simulink model "c00011M_harness"  (R2018a)
settings: Solver=FixedStepAuto  StartTime=0.0  StopTime=300  FixedStep=0.1  RelTol=1e-3
undefined symbols (not defined in the file): A1, hmax, PriorityTank, R1, R2, sigbuilder_block
(part 20 of 73)

== system c00011M_harness/M164/Tank3 ==
  CT3 : Inport
  F3 : Inport  Port=2
  E3 : Inport  Port=3
  T3 : Inport  Port=4
  EB3 : Inport  Port=5
  LL1 : Inport  Port=6
  LL2 : Inport  Port=7
  Control : Subsystem
  Logical Operator : Logic  AllPortsSameDT=off  OutDataTypeStr=boolean
  MasterTankControl : Subsystem
  Memory : Memory
  Memory1 : Memory
  Memory2 : Memory
  TankModel : Subsystem
  LL3 : Outport
  wires:
  TankModel/1(LiquidLevel) -> Memory/1, LL3/1
  Control/1(LiquidIn) -> Logical Operator/1
  Control/2(LiquidOut) -> TankModel/2(LiquidOut)
  Memory/1 -> MasterTankControl/3(LiquidTank3), Control/5(LiquidLevel)
  CT3/1 -> Control/1(ControlType)
  F3/1 -> Control/2(Fill)
  E3/1 -> Control/3(Empty)
  LL2/1 -> Memory2/1
  Memory2/1 -> MasterTankControl/2(LiquidTank2)
  Memory1/1 -> MasterTankControl/1(LiquidTank1)
  EB3/1 -> Control/4(EmergencyButton)
  MasterTankControl/1(AllowTheTankFilling) -> Logical Operator/2
  Logical Operator/1 -> TankModel/1(LiquidIn)
  LL1/1 -> Memory1/1

== system c00011M_harness/M165/Tank1 ==
  CT1 : Inport
  MR1 : Inport  Port=2
  T1 : Inport  Port=3
  EB1 : Inport  Port=4
  LL2 : Inport  Port=5
  LL3 : Inport  Port=6
  Control : Subsystem
  Logical Operator : Logic  AllPortsSameDT=off  OutDataTypeStr=boolean
  MasterTankControl : Subsystem
  Memory : Memory
  Memory1 : Memory
  Memory2 : Memory
  TankModel : Subsystem
  LL1 : Outport
  wires:
  TankModel/1(LiquidLevel) -> Memory/1, LL1/1
  Control/1(LiquidIn) -> Logical Operator/1
  Control/2(LiquidOut) -> TankModel/2(LiquidOut)
  Memory/1 -> Control/5(LiquidLevel), MasterTankControl/1(LiquidTank1)
  MR1/1 -> Control/3(ManualReference)
  CT1/1 -> Control/2(StartMaintenance), Control/1(ControlType)
  LL3/1 -> Memory2/1
  Memory2/1 -> MasterTankControl/3(LiquidTank3)
  Memory1/1 -> MasterTankControl/2(LiquidTank2)
  EB1/1 -> Control/4(EmergencyButton)
  MasterTankControl/1(AllowTheTankFilling) -> Logical Operator/2
  Logical Operator/1 -> TankModel/1(LiquidIn)
  LL2/1 -> Memory1/1

== system c00011M_harness/M165/Tank2 ==
  CT2 : Inport
  MR2 : Inport  Port=2
  T2 : Inport  Port=3
  EB2 : Inport  Port=4
  LL1 : Inport  Port=5
  LL3 : Inport  Port=6
  Control : Subsystem
  Logical Operator : Logic  AllPortsSameDT=off  OutDataTypeStr=boolean
  MasterTankControl : Subsystem
  Memory : Memory
  Memory1 : Memory
  Memory2 : Memory
  TankModel : Subsystem
  LL2 : Outport
  wires:
  TankModel/1(LiquidLevel) -> Memory/1, LL2/1
  Control/1(LiquidIn) -> Logical Operator/1
  Control/2(LiquidOut) -> TankModel/2(LiquidOut)
  Memory/1 -> Control/5(LiquidLevel), MasterTankControl/2(LiquidTank2)
  MR2/1 -> Control/3(ManualReference)
  CT2/1 -> Control/2(StartMaintenance), Control/1(ControlType)
  LL3/1 -> Memory2/1
  Memory2/1 -> MasterTankControl/3(LiquidTank3)
  Memory1/1 -> MasterTankControl/1(LiquidTank1)
  EB2/1 -> Control/4(EmergencyButton)
  MasterTankControl/1(AllowTheTankFilling) -> Logical Operator/2
  Logical Operator/1 -> TankModel/1(LiquidIn)
  LL1/1 -> Memory1/1

== system c00011M_harness/M165/Tank3 ==
  CT3 : Inport
  F3 : Inport  Port=2
  E3 : Inport  Port=3
  T3 : Inport  Port=4
  EB3 : Inport  Port=5
  LL1 : Inport  Port=6
  LL2 : Inport  Port=7
  Control : Subsystem
  Logical Operator : Logic  AllPortsSameDT=off  OutDataTypeStr=boolean
  MasterTankControl : Subsystem
  Memory : Memory
  Memory1 : Memory
  Memory2 : Memory
  TankModel : Subsystem
  LL3 : Outport
  wires:
  TankModel/1(LiquidLevel) -> Memory/1, LL3/1
  Control/1(LiquidIn) -> Logical Operator/1
  Control/2(LiquidOut) -> TankModel/2(LiquidOut)
  Memory/1 -> MasterTankControl/3(LiquidTank3), Control/5(LiquidLevel)
  CT3/1 -> Control/1(ControlType)
  F3/1 -> Control/2(Fill)
  E3/1 -> Control/3(Empty)
  LL2/1 -> Memory2/1
  Memory2/1 -> MasterTankControl/2(LiquidTank2)
  Memory1/1 -> MasterTankControl/1(LiquidTank1)
  EB3/1 -> Control/4(EmergencyButton)
  MasterTankControl/1(AllowTheTankFilling) -> Logical Operator/2
  Logical Operator/1 -> TankModel/1(LiquidIn)
  LL1/1 -> Memory1/1

== system c00011M_harness/M200/Tank1 ==
  CT1 : Inport
  MR1 : Inport  Port=2
  T1 : Inport  Port=3
  EB1 : Inport  Port=4
  LL2 : Inport  Port=5
  LL3 : Inport  Port=6
  Control : Subsystem
  Logical Operator : Logic  AllPortsSameDT=off  OutDataTypeStr=boolean
  MasterTankControl : Subsystem
  Memory : Memory
  Memory1 : Memory
  Memory2 : Memory
  TankModel : Subsystem
  LL1 : Outport
  wires:
  TankModel/1(LiquidLevel) -> Memory/1, LL1/1
  Control/1(LiquidIn) -> Logical Operator/1
  Control/2(LiquidOut) -> TankModel/2(LiquidOut)
  Memory/1 -> Control/5(LiquidLevel), MasterTankControl/1(LiquidTank1)
  MR1/1 -> Control/3(ManualReference)
  CT1/1 -> Control/2(StartMaintenance), Control/1(ControlType)
  LL3/1 -> Memory2/1
  Memory2/1 -> MasterTankControl/3(LiquidTank3)
  Memory1/1 -> MasterTankControl/2(LiquidTank2)
  EB1/1 -> Control/4(EmergencyButton)
  MasterTankControl/1(AllowTheTankFilling) -> Logical Operator/2
  Logical Operator/1 -> TankModel/1(LiquidIn)
  LL2/1 -> Memory1/1

== system c00011M_harness/M200/Tank2 ==
  CT2 : Inport
  MR2 : Inport  Port=2
  T2 : Inport  Port=3
  EB2 : Inport  Port=4
  LL1 : Inport  Port=5
  LL3 : Inport  Port=6
  Control : Subsystem
  Logical Operator : Logic  AllPortsSameDT=off  OutDataTypeStr=boolean
  MasterTankControl : Subsystem
  Memory : Memory
  Memory1 : Memory
  Memory2 : Memory
  TankModel : Subsystem
  LL2 : Outport
  wires:
  TankModel/1(LiquidLevel) -> Memory/1, LL2/1
  Control/1(LiquidIn) -> Logical Operator/1
  Control/2(LiquidOut) -> TankModel/2(LiquidOut)
  Memory/1 -> Control/5(LiquidLevel), MasterTankControl/2(LiquidTank2)
  MR2/1 -> Control/3(ManualReference)
  CT2/1 -> Control/2(StartMaintenance), Control/1(ControlType)
  LL3/1 -> Memory2/1
  Memory2/1 -> MasterTankControl/3(LiquidTank3)
  Memory1/1 -> MasterTankControl/1(LiquidTank1)
  EB2/1 -> Control/4(EmergencyButton)
  MasterTankControl/1(AllowTheTankFilling) -> Logical Operator/2
  Logical Operator/1 -> TankModel/1(LiquidIn)
  LL1/1 -> Memory1/1

== system c00011M_harness/M200/Tank3 ==
  CT3 : Inport
  F3 : Inport  Port=2
  E3 : Inport  Port=3
  T3 : Inport  Port=4
  EB3 : Inport  Port=5
  LL1 : Inport  Port=6
  LL2 : Inport  Port=7
  Control : Subsystem
  Logical Operator : Logic  AllPortsSameDT=off  OutDataTypeStr=boolean
  MasterTankControl : Subsystem
  Memory : Memory
  Memory1 : Memory
  Memory2 : Memory
  TankModel : Subsystem
  LL3 : Outport
  wires:
  TankModel/1(LiquidLevel) -> Memory/1, LL3/1
  Control/1(LiquidIn) -> Logical Operator/1
  Control/2(LiquidOut) -> TankModel/2(LiquidOut)
  Memory/1 -> MasterTankControl/3(LiquidTank3), Control/5(LiquidLevel)
  CT3/1 -> Control/1(ControlType)
  F3/1 -> Control/2(Fill)
  E3/1 -> Control/3(Empty)
  LL2/1 -> Memory2/1
  Memory2/1 -> MasterTankControl/2(LiquidTank2)
  Memory1/1 -> MasterTankControl/1(LiquidTank1)
  EB3/1 -> Control/4(EmergencyButton)
  MasterTankControl/1(AllowTheTankFilling) -> Logical Operator/2
  Logical Operator/1 -> TankModel/1(LiquidIn)
  LL1/1 -> Memory1/1

== system c00011M_harness/M201/Tank1 ==
  CT1 : Inport
  MR1 : Inport  Port=2
  T1 : Inport  Port=3
  EB1 : Inport  Port=4
  LL2 : Inport  Port=5
  LL3 : Inport  Port=6
  Control : Subsystem
  Logical Operator : Logic  AllPortsSameDT=off  OutDataTypeStr=boolean
  MasterTankControl : Subsystem
  Memory : Memory
  Memory1 : Memory
  Memory2 : Memory
  TankModel : Subsystem
  LL1 : Outport
  wires:
  TankModel/1(LiquidLevel) -> Memory/1, LL1/1
  Control/1(LiquidIn) -> Logical Operator/1
  Control/2(LiquidOut) -> TankModel/2(LiquidOut)
  Memory/1 -> Control/5(LiquidLevel), MasterTankControl/1(LiquidTank1)
  MR1/1 -> Control/3(ManualReference)
  CT1/1 -> Control/2(StartMaintenance), Control/1(ControlType)
  LL3/1 -> Memory2/1
  Memory2/1 -> MasterTankControl/3(LiquidTank3)
  Memory1/1 -> MasterTankControl/2(LiquidTank2)
  EB1/1 -> Control/4(EmergencyButton)
  MasterTankControl/1(AllowTheTankFilling) -> Logical Operator/2
  Logical Operator/1 -> TankModel/1(LiquidIn)
  LL2/1 -> Memory1/1

== system c00011M_harness/M201/Tank2 ==
  CT2 : Inport
  MR2 : Inport  Port=2
  T2 : Inport  Port=3
  EB2 : Inport  Port=4
  LL1 : Inport  Port=5
  LL3 : Inport  Port=6
  Control : Subsystem
  Logical Operator : Logic  AllPortsSameDT=off  OutDataTypeStr=boolean
  MasterTankControl : Subsystem
  Memory : Memory
  Memory1 : Memory
  Memory2 : Memory
  TankModel : Subsystem
  LL2 : Outport
  wires:
  TankModel/1(LiquidLevel) -> Memory/1, LL2/1
  Control/1(LiquidIn) -> Logical Operator/1
  Control/2(LiquidOut) -> TankModel/2(LiquidOut)
  Memory/1 -> Control/5(LiquidLevel), MasterTankControl/2(LiquidTank2)
  MR2/1 -> Control/3(ManualReference)
  CT2/1 -> Control/2(StartMaintenance), Control/1(ControlType)
  LL3/1 -> Memory2/1
  Memory2/1 -> MasterTankControl/3(LiquidTank3)
  Memory1/1 -> MasterTankControl/1(LiquidTank1)
  EB2/1 -> Control/4(EmergencyButton)
  MasterTankControl/1(AllowTheTankFilling) -> Logical Operator/2
  Logical Operator/1 -> TankModel/1(LiquidIn)
  LL1/1 -> Memory1/1

== system c00011M_harness/M201/Tank3 ==
  CT3 : Inport
  F3 : Inport  Port=2
  E3 : Inport  Port=3
  T3 : Inport  Port=4
  EB3 : Inport  Port=5
  LL1 : Inport  Port=6
  LL2 : Inport  Port=7
  Control : Subsystem
  Logical Operator : Logic  AllPortsSameDT=off  OutDataTypeStr=boolean
  MasterTankControl : Subsystem
  Memory : Memory
  Memory1 : Memory
  Memory2 : Memory
  TankModel : Subsystem
  LL3 : Outport
  wires:
  TankModel/1(LiquidLevel) -> Memory/1, LL3/1
  Control/1(LiquidIn) -> Logical Operator/1
  Control/2(LiquidOut) -> TankModel/2(LiquidOut)
  Memory/1 -> MasterTankControl/3(LiquidTank3), Control/5(LiquidLevel)
  CT3/1 -> Control/1(ControlType)
  F3/1 -> Control/2(Fill)
  E3/1 -> Control/3(Empty)
  LL2/1 -> Memory2/1
  Memory2/1 -> MasterTankControl/2(LiquidTank2)
  Memory1/1 -> MasterTankControl/1(LiquidTank1)
  EB3/1 -> Control/4(EmergencyButton)
  MasterTankControl/1(AllowTheTankFilling) -> Logical Operator/2
  Logical Operator/1 -> TankModel/1(LiquidIn)
  LL1/1 -> Memory1/1

== system c00011M_harness/M202/Tank1 ==
  CT1 : Inport
  MR1 : Inport  Port=2
  T1 : Inport  Port=3
  EB1 : Inport  Port=4
  LL2 : Inport  Port=5
  LL3 : Inport  Port=6
  Control : Subsystem
  Logical Operator : Logic  AllPortsSameDT=off  OutDataTypeStr=boolean
  MasterTankControl : Subsystem
  Memory : Memory
  Memory1 : Memory
  Memory2 : Memory
  TankModel : Subsystem
  LL1 : Outport
  wires:
  TankModel/1(LiquidLevel) -> Memory/1, LL1/1
  Control/1(LiquidIn) -> Logical Operator/1
  Control/2(LiquidOut) -> TankModel/2(LiquidOut)
  Memory/1 -> Control/5(LiquidLevel), MasterTankControl/1(LiquidTank1)
  MR1/1 -> Control/3(ManualReference)
  CT1/1 -> Control/2(StartMaintenance), Control/1(ControlType)
  LL3/1 -> Memory2/1
  Memory2/1 -> MasterTankControl/3(LiquidTank3)
  Memory1/1 -> MasterTankControl/2(LiquidTank2)
  EB1/1 -> Control/4(EmergencyButton)
  MasterTankControl/1(AllowTheTankFilling) -> Logical Operator/2
  Logical Operator/1 -> TankModel/1(LiquidIn)
  LL2/1 -> Memory1/1

== system c00011M_harness/M202/Tank2 ==
  CT2 : Inport
  MR2 : Inport  Port=2
  T2 : Inport  Port=3
  EB2 : Inport  Port=4
  LL1 : Inport  Port=5
  LL3 : Inport  Port=6
  Control : Subsystem
  Logical Operator : Logic  AllPortsSameDT=off  OutDataTypeStr=boolean
  MasterTankControl : Subsystem
  Memory : Memory
  Memory1 : Memory
  Memory2 : Memory
  TankModel : Subsystem
  LL2 : Outport
  wires:
  TankModel/1(LiquidLevel) -> Memory/1, LL2/1
  Control/1(LiquidIn) -> Logical Operator/1
  Control/2(LiquidOut) -> TankModel/2(LiquidOut)
  Memory/1 -> Control/5(LiquidLevel), MasterTankControl/2(LiquidTank2)
  MR2/1 -> Control/3(ManualReference)
  CT2/1 -> Control/2(StartMaintenance), Control/1(ControlType)
  LL3/1 -> Memory2/1
  Memory2/1 -> MasterTankControl/3(LiquidTank3)
  Memory1/1 -> MasterTankControl/1(LiquidTank1)
  EB2/1 -> Control/4(EmergencyButton)
  MasterTankControl/1(AllowTheTankFilling) -> Logical Operator/2
  Logical Operator/1 -> TankModel/1(LiquidIn)
  LL1/1 -> Memory1/1

== system c00011M_harness/M202/Tank3 ==
  CT3 : Inport
  F3 : Inport  Port=2
  E3 : Inport  Port=3
  T3 : Inport  Port=4
  EB3 : Inport  Port=5
  LL1 : Inport  Port=6
  LL2 : Inport  Port=7
  Control : Subsystem
  Logical Operator : Logic  AllPortsSameDT=off  OutDataTypeStr=boolean
  MasterTankControl : Subsystem
  Memory : Memory
  Memory1 : Memory
  Memory2 : Memory
  TankModel : Subsystem
  LL3 : Outport
  wires:
  TankModel/1(LiquidLevel) -> Memory/1, LL3/1
  Control/1(LiquidIn) -> Logical Operator/1
  Control/2(LiquidOut) -> TankModel/2(LiquidOut)
  Memory/1 -> MasterTankControl/3(LiquidTank3), Control/5(LiquidLevel)
  CT3/1 -> Control/1(ControlType)
  F3/1 -> Control/2(Fill)
  E3/1 -> Control/3(Empty)
  LL2/1 -> Memory2/1
  Memory2/1 -> MasterTankControl/2(LiquidTank2)
  Memory1/1 -> MasterTankControl/1(LiquidTank1)
  EB3/1 -> Control/4(EmergencyButton)
  MasterTankControl/1(AllowTheTankFilling) -> Logical Operator/2
  Logical Operator/1 -> TankModel/1(LiquidIn)
  LL1/1 -> Memory1/1

== system c00011M_harness/M203/Tank1 ==
  CT1 : Inport
  MR1 : Inport  Port=2
  T1 : Inport  Port=3
  EB1 : Inport  Port=4
  LL2 : Inport  Port=5
  LL3 : Inport  Port=6
  Control : Subsystem
  Logical Operator : Logic  AllPortsSameDT=off  OutDataTypeStr=boolean
  MasterTankControl : Subsystem
  Memory : Memory
  Memory1 : Memory
  Memory2 : Memory
  TankModel : Subsystem
  LL1 : Outport
  wires:
  TankModel/1(LiquidLevel) -> Memory/1, LL1/1
  Control/1(LiquidIn) -> Logical Operator/1
  Control/2(LiquidOut) -> TankModel/2(LiquidOut)
  Memory/1 -> Control/5(LiquidLevel), MasterTankControl/1(LiquidTank1)
  MR1/1 -> Control/3(ManualReference)
  CT1/1 -> Control/2(StartMaintenance), Control/1(ControlType)
  LL3/1 -> Memory2/1
  Memory2/1 -> MasterTankControl/3(LiquidTank3)
  Memory1/1 -> MasterTankControl/2(LiquidTank2)
  EB1/1 -> Control/4(EmergencyButton)
  MasterTankControl/1(AllowTheTankFilling) -> Logical Operator/2
  Logical Operator/1 -> TankModel/1(LiquidIn)
  LL2/1 -> Memory1/1

== system c00011M_harness/M203/Tank2 ==
  CT2 : Inport
  MR2 : Inport  Port=2
  T2 : Inport  Port=3
  EB2 : Inport  Port=4
  LL1 : Inport  Port=5
  LL3 : Inport  Port=6
  Control : Subsystem
  Logical Operator : Logic  AllPortsSameDT=off  OutDataTypeStr=boolean
  MasterTankControl : Subsystem
  Memory : Memory
  Memory1 : Memory
  Memory2 : Memory
  TankModel : Subsystem
  LL2 : Outport
  wires:
  TankModel/1(LiquidLevel) -> Memory/1, LL2/1
  Control/1(LiquidIn) -> Logical Operator/1
  Control/2(LiquidOut) -> TankModel/2(LiquidOut)
  Memory/1 -> Control/5(LiquidLevel), MasterTankControl/2(LiquidTank2)
  MR2/1 -> Control/3(ManualReference)
  CT2/1 -> Control/2(StartMaintenance), Control/1(ControlType)
  LL3/1 -> Memory2/1
  Memory2/1 -> MasterTankControl/3(LiquidTank3)
  Memory1/1 -> MasterTankControl/1(LiquidTank1)
  EB2/1 -> Control/4(EmergencyButton)
  MasterTankControl/1(AllowTheTankFilling) -> Logical Operator/2
  Logical Operator/1 -> TankModel/1(LiquidIn)
  LL1/1 -> Memory1/1

== system c00011M_harness/M203/Tank3 ==
  CT3 : Inport
  F3 : Inport  Port=2
  E3 : Inport  Port=3
  T3 : Inport  Port=4
  EB3 : Inport  Port=5
  LL1 : Inport  Port=6
  LL2 : Inport  Port=7
  Control : Subsystem
  Logical Operator : Logic  AllPortsSameDT=off  OutDataTypeStr=boolean
  MasterTankControl : Subsystem
  Memory : Memory
  Memory1 : Memory
  Memory2 : Memory
  TankModel : Subsystem
  LL3 : Outport
  wires:
  TankModel/1(LiquidLevel) -> Memory/1, LL3/1
  Control/1(LiquidIn) -> Logical Operator/1
  Control/2(LiquidOut) -> TankModel/2(LiquidOut)
  Memory/1 -> MasterTankControl/3(LiquidTank3), Control/5(LiquidLevel)
  CT3/1 -> Control/1(ControlType)
  F3/1 -> Control/2(Fill)
  E3/1 -> Control/3(Empty)
  LL2/1 -> Memory2/1
  Memory2/1 -> MasterTankControl/2(LiquidTank2)
  Memory1/1 -> MasterTankControl/1(LiquidTank1)
  EB3/1 -> Control/4(EmergencyButton)
  MasterTankControl/1(AllowTheTankFilling) -> Logical Operator/2
  Logical Operator/1 -> TankModel/1(LiquidIn)
  LL1/1 -> Memory1/1

== system c00011M_harness/M204/Tank1 ==
  CT1 : Inport
  MR1 : Inport  Port=2
  T1 : Inport  Port=3
  EB1 : Inport  Port=4
  LL2 : Inport  Port=5
  LL3 : Inport  Port=6
  Control : Subsystem
  Logical Operator : Logic  AllPortsSameDT=off  OutDataTypeStr=boolean
  MasterTankControl : Subsystem
  Memory : Memory
  Memory1 : Memory
  Memory2 : Memory
  TankModel : Subsystem
  LL1 : Outport
  wires:
  TankModel/1(LiquidLevel) -> Memory/1, LL1/1
  Control/1(LiquidIn) -> Logical Operator/1
  Control/2(LiquidOut) -> TankModel/2(LiquidOut)
  Memory/1 -> Control/5(LiquidLevel), MasterTankControl/1(LiquidTank1)
  MR1/1 -> Control/3(ManualReference)
  CT1/1 -> Control/2(StartMaintenance), Control/1(ControlType)
  LL3/1 -> Memory2/1
  Memory2/1 -> MasterTankControl/3(LiquidTank3)
  Memory1/1 -> MasterTankControl/2(LiquidTank2)
  EB1/1 -> Control/4(EmergencyButton)
  MasterTankControl/1(AllowTheTankFilling) -> Logical Operator/2
  Logical Operator/1 -> TankModel/1(LiquidIn)
  LL2/1 -> Memory1/1

== system c00011M_harness/M204/Tank2 ==
  CT2 : Inport
  MR2 : Inport  Port=2
  T2 : Inport  Port=3
  EB2 : Inport  Port=4
  LL1 : Inport  Port=5
  LL3 : Inport  Port=6
  Control : Subsystem
  Logical Operator : Logic  AllPortsSameDT=off  OutDataTypeStr=boolean
  MasterTankControl : Subsystem
  Memory : Memory
  Memory1 : Memory
  Memory2 : Memory
  TankModel : Subsystem
  LL2 : Outport
  wires:
  TankModel/1(LiquidLevel) -> Memory/1, LL2/1
  Control/1(LiquidIn) -> Logical Operator/1
  Control/2(LiquidOut) -> TankModel/2(LiquidOut)
  Memory/1 -> Control/5(LiquidLevel), MasterTankControl/2(LiquidTank2)
  MR2/1 -> Control/3(ManualReference)
  CT2/1 -> Control/2(StartMaintenance), Control/1(ControlType)
  LL3/1 -> Memory2/1
  Memory2/1 -> MasterTankControl/3(LiquidTank3)
  Memory1/1 -> MasterTankControl/1(LiquidTank1)
  EB2/1 -> Control/4(EmergencyButton)
  MasterTankControl/1(AllowTheTankFilling) -> Logical Operator/2
  Logical Operator/1 -> TankModel/1(LiquidIn)
  LL1/1 -> Memory1/1

== system c00011M_harness/M204/Tank3 ==
  CT3 : Inport
  F3 : Inport  Port=2
  E3 : Inport  Port=3
  T3 : Inport  Port=4
  EB3 : Inport  Port=5
  LL1 : Inport  Port=6
  LL2 : Inport  Port=7
  Control : Subsystem
  Logical Operator : Logic  AllPortsSameDT=off  OutDataTypeStr=boolean
  MasterTankControl : Subsystem
  Memory : Memory
  Memory1 : Memory
  Memory2 : Memory
  TankModel : Subsystem
  LL3 : Outport
  wires:
  TankModel/1(LiquidLevel) -> Memory/1, LL3/1
  Control/1(LiquidIn) -> Logical Operator/1
  Control/2(LiquidOut) -> TankModel/2(LiquidOut)
  Memory/1 -> MasterTankControl/3(LiquidTank3), Control/5(LiquidLevel)
  CT3/1 -> Control/1(ControlType)
  F3/1 -> Control/2(Fill)
  E3/1 -> Control/3(Empty)
  LL2/1 -> Memory2/1
  Memory2/1 -> MasterTankControl/2(LiquidTank2)
  Memory1/1 -> MasterTankControl/1(LiquidTank1)
  EB3/1 -> Control/4(EmergencyButton)
  MasterTankControl/1(AllowTheTankFilling) -> Logical Operator/2
  Logical Operator/1 -> TankModel/1(LiquidIn)
  LL1/1 -> Memory1/1

== system c00011M_harness/M205/Tank1 ==
  CT1 : Inport
  MR1 : Inport  Port=2
  T1 : Inport  Port=3
  EB1 : Inport  Port=4
  LL2 : Inport  Port=5
  LL3 : Inport  Port=6
  Control : Subsystem
  Logical Operator : Logic  AllPortsSameDT=off  OutDataTypeStr=boolean
  MasterTankControl : Subsystem
  Memory : Memory
  Memory1 : Memory
  Memory2 : Memory
  TankModel : Subsystem
  LL1 : Outport
  wires:
  TankModel/1(LiquidLevel) -> Memory/1, LL1/1
  Control/1(LiquidIn) -> Logical Operator/1
  Control/2(LiquidOut) -> TankModel/2(LiquidOut)
  Memory/1 -> Control/5(LiquidLevel), MasterTankControl/1(LiquidTank1)
  MR1/1 -> Control/3(ManualReference)
  CT1/1 -> Control/2(StartMaintenance), Control/1(ControlType)
  LL3/1 -> Memory2/1
  Memory2/1 -> MasterTankControl/3(LiquidTank3)
  Memory1/1 -> MasterTankControl/2(LiquidTank2)
  EB1/1 -> Control/4(EmergencyButton)
  MasterTankControl/1(AllowTheTankFilling) -> Logical Operator/2
  Logical Operator/1 -> TankModel/1(LiquidIn)
  LL2/1 -> Memory1/1

== system c00011M_harness/M205/Tank2 ==
  CT2 : Inport
  MR2 : Inport  Port=2
  T2 : Inport  Port=3
  EB2 : Inport  Port=4
  LL1 : Inport  Port=5
  LL3 : Inport  Port=6
  Control : Subsystem
  Logical Operator : Logic  AllPortsSameDT=off  OutDataTypeStr=boolean
  MasterTankControl : Subsystem
  Memory : Memory
  Memory1 : Memory
  Memory2 : Memory
  TankModel : Subsystem
  LL2 : Outport
  wires:
  TankModel/1(LiquidLevel) -> Memory/1, LL2/1
  Control/1(LiquidIn) -> Logical Operator/1
  Control/2(LiquidOut) -> TankModel/2(LiquidOut)
  Memory/1 -> Control/5(LiquidLevel), MasterTankControl/2(LiquidTank2)
  MR2/1 -> Control/3(ManualReference)
  CT2/1 -> Control/2(StartMaintenance), Control/1(ControlType)
  LL3/1 -> Memory2/1
  Memory2/1 -> MasterTankControl/3(LiquidTank3)
  Memory1/1 -> MasterTankControl/1(LiquidTank1)
  EB2/1 -> Control/4(EmergencyButton)
  MasterTankControl/1(AllowTheTankFilling) -> Logical Operator/2
  Logical Operator/1 -> TankModel/1(LiquidIn)
  LL1/1 -> Memory1/1

== system c00011M_harness/M205/Tank3 ==
  CT3 : Inport
  F3 : Inport  Port=2
  E3 : Inport  Port=3
  T3 : Inport  Port=4
  EB3 : Inport  Port=5
  LL1 : Inport  Port=6
  LL2 : Inport  Port=7
  Control : Subsystem
  Logical Operator : Logic  AllPortsSameDT=off  OutDataTypeStr=boolean
  MasterTankControl : Subsystem
  Memory : Memory
  Memory1 : Memory
  Memory2 : Memory
  TankModel : Subsystem
  LL3 : Outport
  wires:
  TankModel/1(LiquidLevel) -> Memory/1, LL3/1
  Control/1(LiquidIn) -> Logical Operator/1
  Control/2(LiquidOut) -> TankModel/2(LiquidOut)
  Memory/1 -> MasterTankControl/3(LiquidTank3), Control/5(LiquidLevel)
  CT3/1 -> Control/1(ControlType)
  F3/1 -> Control/2(Fill)
  E3/1 -> Control/3(Empty)
  LL2/1 -> Memory2/1
  Memory2/1 -> MasterTankControl/2(LiquidTank2)
  Memory1/1 -> MasterTankControl/1(LiquidTank1)
  EB3/1 -> Control/4(EmergencyButton)
  MasterTankControl/1(AllowTheTankFilling) -> Logical Operator/2
  Logical Operator/1 -> TankModel/1(LiquidIn)
  LL1/1 -> Memory1/1

== system c00011M_harness/M206/Tank1 ==
  CT1 : Inport
  MR1 : Inport  Port=2
  T1 : Inport  Port=3
  EB1 : Inport  Port=4
  LL2 : Inport  Port=5
  LL3 : Inport  Port=6
  Control : Subsystem
  Logical Operator : Logic  AllPortsSameDT=off  OutDataTypeStr=boolean
  MasterTankControl : Subsystem
  Memory : Memory
  Memory1 : Memory
  Memory2 : Memory
  TankModel : Subsystem
  LL1 : Outport
  wires:
  TankModel/1(LiquidLevel) -> Memory/1, LL1/1
  Control/1(LiquidIn) -> Logical Operator/1
  Control/2(LiquidOut) -> TankModel/2(LiquidOut)
  Memory/1 -> Control/5(LiquidLevel), MasterTankControl/1(LiquidTank1)
  MR1/1 -> Control/3(ManualReference)
  CT1/1 -> Control/2(StartMaintenance), Control/1(ControlType)
  LL3/1 -> Memory2/1
  Memory2/1 -> MasterTankControl/3(LiquidTank3)
  Memory1/1 -> MasterTankControl/2(LiquidTank2)
  EB1/1 -> Control/4(EmergencyButton)
  MasterTankControl/1(AllowTheTankFilling) -> Logical Operator/2
  Logical Operator/1 -> TankModel/1(LiquidIn)
  LL2/1 -> Memory1/1

== system c00011M_harness/M206/Tank2 ==
  CT2 : Inport
  MR2 : Inport  Port=2
  T2 : Inport  Port=3
  EB2 : Inport  Port=4
  LL1 : Inport  Port=5
  LL3 : Inport  Port=6
  Control : Subsystem
  Logical Operator : Logic  AllPortsSameDT=off  OutDataTypeStr=boolean
  MasterTankControl : Subsystem
  Memory : Memory
  Memory1 : Memory
  Memory2 : Memory
  TankModel : Subsystem
  LL2 : Outport
  wires:
  TankModel/1(LiquidLevel) -> Memory/1, LL2/1
  Control/1(LiquidIn) -> Logical Operator/1
  Control/2(LiquidOut) -> TankModel/2(LiquidOut)
  Memory/1 -> Control/5(LiquidLevel), MasterTankControl/2(LiquidTank2)
  MR2/1 -> Control/3(ManualReference)
  CT2/1 -> Control/2(StartMaintenance), Control/1(ControlType)
  LL3/1 -> Memory2/1
  Memory2/1 -> MasterTankControl/3(LiquidTank3)
  Memory1/1 -> MasterTankControl/1(LiquidTank1)
  EB2/1 -> Control/4(EmergencyButton)
  MasterTankControl/1(AllowTheTankFilling) -> Logical Operator/2
  Logical Operator/1 -> TankModel/1(LiquidIn)
  LL1/1 -> Memory1/1

== system c00011M_harness/M206/Tank3 ==
  CT3 : Inport
  F3 : Inport  Port=2
  E3 : Inport  Port=3
  T3 : Inport  Port=4
  EB3 : Inport  Port=5
  LL1 : Inport  Port=6
  LL2 : Inport  Port=7
  Control : Subsystem
  Logical Operator : Logic  AllPortsSameDT=off  OutDataTypeStr=boolean
  MasterTankControl : Subsystem
  Memory : Memory
  Memory1 : Memory
  Memory2 : Memory
  TankModel : Subsystem
  LL3 : Outport
  wires:
  TankModel/1(LiquidLevel) -> Memory/1, LL3/1
  Control/1(LiquidIn) -> Logical Operator/1
  Control/2(LiquidOut) -> TankModel/2(LiquidOut)
  Memory/1 -> MasterTankControl/3(LiquidTank3), Control/5(LiquidLevel)
  CT3/1 -> Control/1(ControlType)
  F3/1 -> Control/2(Fill)
  E3/1 -> Control/3(Empty)
  LL2/1 -> Memory2/1
  Memory2/1 -> MasterTankControl/2(LiquidTank2)
  Memory1/1 -> MasterTankControl/1(LiquidTank1)
  EB3/1 -> Control/4(EmergencyButton)
  MasterTankControl/1(AllowTheTankFilling) -> Logical Operator/2
  Logical Operator/1 -> TankModel/1(LiquidIn)
  LL1/1 -> Memory1/1

== system c00011M_harness/M207/Tank1 ==
  CT1 : Inport
  MR1 : Inport  Port=2
  T1 : Inport  Port=3
  EB1 : Inport  Port=4
  LL2 : Inport  Port=5
  LL3 : Inport  Port=6
  Control : Subsystem
  Logical Operator : Logic  AllPortsSameDT=off  OutDataTypeStr=boolean
  MasterTankControl : Subsystem
  Memory : Memory
  Memory1 : Memory
  Memory2 : Memory
  TankModel : Subsystem
  LL1 : Outport
  wires:
  TankModel/1(LiquidLevel) -> Memory/1, LL1/1
  Control/1(LiquidIn) -> Logical Operator/1
  Control/2(LiquidOut) -> TankModel/2(LiquidOut)
  Memory/1 -> Control/5(LiquidLevel), MasterTankControl/1(LiquidTank1)
  MR1/1 -> Control/3(ManualReference)
  CT1/1 -> Control/2(StartMaintenance), Control/1(ControlType)
  LL3/1 -> Memory2/1
  Memory2/1 -> MasterTankControl/3(LiquidTank3)
  Memory1/1 -> MasterTankControl/2(LiquidTank2)
  EB1/1 -> Control/4(EmergencyButton)
  MasterTankControl/1(AllowTheTankFilling) -> Logical Operator/2
  Logical Operator/1 -> TankModel/1(LiquidIn)
  LL2/1 -> Memory1/1

== system c00011M_harness/M207/Tank2 ==
  CT2 : Inport
  MR2 : Inport  Port=2
  T2 : Inport  Port=3
  EB2 : Inport  Port=4
  LL1 : Inport  Port=5
  LL3 : Inport  Port=6
  Control : Subsystem
  Logical Operator : Logic  AllPortsSameDT=off  OutDataTypeStr=boolean
  MasterTankControl : Subsystem
  Memory : Memory
  Memory1 : Memory
  Memory2 : Memory
  TankModel : Subsystem
  LL2 : Outport
  wires:
  TankModel/1(LiquidLevel) -> Memory/1, LL2/1
  Control/1(LiquidIn) -> Logical Operator/1
  Control/2(LiquidOut) -> TankModel/2(LiquidOut)
  Memory/1 -> Control/5(LiquidLevel), MasterTankControl/2(LiquidTank2)
  MR2/1 -> Control/3(ManualReference)
  CT2/1 -> Control/2(StartMaintenance), Control/1(ControlType)
  LL3/1 -> Memory2/1
  Memory2/1 -> MasterTankControl/3(LiquidTank3)
  Memory1/1 -> MasterTankControl/1(LiquidTank1)
  EB2/1 -> Control/4(EmergencyButton)
  MasterTankControl/1(AllowTheTankFilling) -> Logical Operator/2
  Logical Operator/1 -> TankModel/1(LiquidIn)
  LL1/1 -> Memory1/1

== system c00011M_harness/M207/Tank3 ==
  CT3 : Inport
  F3 : Inport  Port=2
  E3 : Inport  Port=3
  T3 : Inport  Port=4
  EB3 : Inport  Port=5
  LL1 : Inport  Port=6
  LL2 : Inport  Port=7
  Control : Subsystem
  Logical Operator : Logic  AllPortsSameDT=off  OutDataTypeStr=boolean
  MasterTankControl : Subsystem
  Memory : Memory
  Memory1 : Memory
  Memory2 : Memory
  TankModel : Subsystem
  LL3 : Outport
  wires:
  TankModel/1(LiquidLevel) -> Memory/1, LL3/1
  Control/1(LiquidIn) -> Logical Operator/1
  Control/2(LiquidOut) -> TankModel/2(LiquidOut)
  Memory/1 -> MasterTankControl/3(LiquidTank3), Control/5(LiquidLevel)
  CT3/1 -> Control/1(ControlType)
  F3/1 -> Control/2(Fill)
  E3/1 -> Control/3(Empty)
  LL2/1 -> Memory2/1
  Memory2/1 -> MasterTankControl/2(LiquidTank2)
  Memory1/1 -> MasterTankControl/1(LiquidTank1)
  EB3/1 -> Control/4(EmergencyButton)
  MasterTankControl/1(AllowTheTankFilling) -> Logical Operator/2
  Logical Operator/1 -> TankModel/1(LiquidIn)
  LL1/1 -> Memory1/1

== system c00011M_harness/M208/Tank1 ==
  CT1 : Inport
  MR1 : Inport  Port=2
  T1 : Inport  Port=3
  EB1 : Inport  Port=4
  LL2 : Inport  Port=5
  LL3 : Inport  Port=6
  Control : Subsystem
  Logical Operator : Logic  AllPortsSameDT=off  OutDataTypeStr=boolean
  MasterTankControl : Subsystem
  Memory : Memory
  Memory1 : Memory
  Memory2 : Memory
  TankModel : Subsystem
  LL1 : Outport
  wires:
  TankModel/1(LiquidLevel) -> Memory/1, LL1/1
  Control/1(LiquidIn) -> Logical Operator/1
  Control/2(LiquidOut) -> TankModel/2(LiquidOut)
  Memory/1 -> Control/5(LiquidLevel), MasterTankControl/1(LiquidTank1)
  MR1/1 -> Control/3(ManualReference)
  CT1/1 -> Control/2(StartMaintenance), Control/1(ControlType)
  LL3/1 -> Memory2/1
  Memory2/1 -> MasterTankControl/3(LiquidTank3)
  Memory1/1 -> MasterTankControl/2(LiquidTank2)
  EB1/1 -> Control/4(EmergencyButton)
  MasterTankControl/1(AllowTheTankFilling) -> Logical Operator/2
  Logical Operator/1 -> TankModel/1(LiquidIn)
  LL2/1 -> Memory1/1

== system c00011M_harness/M208/Tank2 ==
  CT2 : Inport
  MR2 : Inport  Port=2
  T2 : Inport  Port=3
  EB2 : Inport  Port=4
  LL1 : Inport  Port=5
  LL3 : Inport  Port=6
  Control : Subsystem
  Logical Operator : Logic  AllPortsSameDT=off  OutDataTypeStr=boolean
  MasterTankControl : Subsystem
  Memory : Memory
  Memory1 : Memory
  Memory2 : Memory
  TankModel : Subsystem
  LL2 : Outport
  wires:
  TankModel/1(LiquidLevel) -> Memory/1, LL2/1
  Control/1(LiquidIn) -> Logical Operator/1
  Control/2(LiquidOut) -> TankModel/2(LiquidOut)
  Memory/1 -> Control/5(LiquidLevel), MasterTankControl/2(LiquidTank2)
  MR2/1 -> Control/3(ManualReference)
  CT2/1 -> Control/2(StartMaintenance), Control/1(ControlType)
  LL3/1 -> Memory2/1
  Memory2/1 -> MasterTankControl/3(LiquidTank3)
  Memory1/1 -> MasterTankControl/1(LiquidTank1)
  EB2/1 -> Control/4(EmergencyButton)
  MasterTankControl/1(AllowTheTankFilling) -> Logical Operator/2
  Logical Operator/1 -> TankModel/1(LiquidIn)
  LL1/1 -> Memory1/1

== system c00011M_harness/M208/Tank3 ==
  CT3 : Inport
  F3 : Inport  Port=2
  E3 : Inport  Port=3
  T3 : Inport  Port=4
  EB3 : Inport  Port=5
  LL1 : Inport  Port=6
  LL2 : Inport  Port=7
  Control : Subsystem
  Logical Operator : Logic  AllPortsSameDT=off  OutDataTypeStr=boolean
  MasterTankControl : Subsystem
  Memory : Memory
  Memory1 : Memory
  Memory2 : Memory
  TankModel : Subsystem
  LL3 : Outport
  wires:
  TankModel/1(LiquidLevel) -> Memory/1, LL3/1
  Control/1(LiquidIn) -> Logical Operator/1
  Control/2(LiquidOut) -> TankModel/2(LiquidOut)
  Memory/1 -> MasterTankControl/3(LiquidTank3), Control/5(LiquidLevel)
  CT3/1 -> Control/1(ControlType)
  F3/1 -> Control/2(Fill)
  E3/1 -> Control/3(Empty)
  LL2/1 -> Memory2/1
  Memory2/1 -> MasterTankControl/2(LiquidTank2)
  Memory1/1 -> MasterTankControl/1(LiquidTank1)
  EB3/1 -> Control/4(EmergencyButton)
  MasterTankControl/1(AllowTheTankFilling) -> Logical Operator/2
  Logical Operator/1 -> TankModel/1(LiquidIn)
  LL1/1 -> Memory1/1

== system c00011M_harness/M209/Tank1 ==
  CT1 : Inport
  MR1 : Inport  Port=2
  T1 : Inport  Port=3
  EB1 : Inport  Port=4
  LL2 : Inport  Port=5
  LL3 : Inport  Port=6
  Control : Subsystem
  Logical Operator : Logic  AllPortsSameDT=off  OutDataTypeStr=boolean
  MasterTankControl : Subsystem
  Memory : Memory
  Memory1 : Memory
  Memory2 : Memory
  TankModel : Subsystem
  LL1 : Outport
  wires:
  TankModel/1(LiquidLevel) -> Memory/1, LL1/1
  Control/1(LiquidIn) -> Logical Operator/1
  Control/2(LiquidOut) -> TankModel/2(LiquidOut)
  Memory/1 -> Control/5(LiquidLevel), MasterTankControl/1(LiquidTank1)
  MR1/1 -> Control/3(ManualReference)
  CT1/1 -> Control/2(StartMaintenance), Control/1(ControlType)
  LL3/1 -> Memory2/1
  Memory2/1 -> MasterTankControl/3(LiquidTank3)
  Memory1/1 -> MasterTankControl/2(LiquidTank2)
  EB1/1 -> Control/4(EmergencyButton)
  MasterTankControl/1(AllowTheTankFilling) -> Logical Operator/2
  Logical Operator/1 -> TankModel/1(LiquidIn)
  LL2/1 -> Memory1/1

== system c00011M_harness/M209/Tank2 ==
  CT2 : Inport
  MR2 : Inport  Port=2
  T2 : Inport  Port=3
  EB2 : Inport  Port=4
  LL1 : Inport  Port=5
  LL3 : Inport  Port=6
  Control : Subsystem
  Logical Operator : Logic  AllPortsSameDT=off  OutDataTypeStr=boolean
  MasterTankControl : Subsystem
  Memory : Memory
  Memory1 : Memory
  Memory2 : Memory
  TankModel : Subsystem
  LL2 : Outport
  wires:
  TankModel/1(LiquidLevel) -> Memory/1, LL2/1
  Control/1(LiquidIn) -> Logical Operator/1
  Control/2(LiquidOut) -> TankModel/2(LiquidOut)
  Memory/1 -> Control/5(LiquidLevel), MasterTankControl/2(LiquidTank2)
  MR2/1 -> Control/3(ManualReference)
  CT2/1 -> Control/2(StartMaintenance), Control/1(ControlType)
  LL3/1 -> Memory2/1
  Memory2/1 -> MasterTankControl/3(LiquidTank3)
  Memory1/1 -> MasterTankControl/1(LiquidTank1)
  EB2/1 -> Control/4(EmergencyButton)
  MasterTankControl/1(AllowTheTankFilling) -> Logical Operator/2
  Logical Operator/1 -> TankModel/1(LiquidIn)
  LL1/1 -> Memory1/1

== system c00011M_harness/M209/Tank3 ==
  CT3 : Inport
  F3 : Inport  Port=2
  E3 : Inport  Port=3
  T3 : Inport  Port=4
  EB3 : Inport  Port=5
  LL1 : Inport  Port=6
  LL2 : Inport  Port=7
  Control : Subsystem
  Logical Operator : Logic  AllPortsSameDT=off  OutDataTypeStr=boolean
  MasterTankControl : Subsystem
  Memory : Memory
  Memory1 : Memory
  Memory2 : Memory
  TankModel : Subsystem
  LL3 : Outport
  wires:
  TankModel/1(LiquidLevel) -> Memory/1, LL3/1
  Control/1(LiquidIn) -> Logical Operator/1
  Control/2(LiquidOut) -> TankModel/2(LiquidOut)
  Memory/1 -> MasterTankControl/3(LiquidTank3), Control/5(LiquidLevel)
  CT3/1 -> Control/1(ControlType)
  F3/1 -> Control/2(Fill)
  E3/1 -> Control/3(Empty)
  LL2/1 -> Memory2/1
  Memory2/1 -> MasterTankControl/2(LiquidTank2)
  Memory1/1 -> MasterTankControl/1(LiquidTank1)
  EB3/1 -> Control/4(EmergencyButton)
  MasterTankControl/1(AllowTheTankFilling) -> Logical Operator/2
  Logical Operator/1 -> TankModel/1(LiquidIn)
  LL1/1 -> Memory1/1

== system c00011M_harness/M222/Tank1 ==
  CT1 : Inport
  MR1 : Inport  Port=2
  T1 : Inport  Port=3
  EB1 : Inport  Port=4
  LL2 : Inport  Port=5
  LL3 : Inport  Port=6
  Control : Subsystem
  Logical Operator : Logic  AllPortsSameDT=off  OutDataTypeStr=boolean
  MasterTankControl : Subsystem
  Memory : Memory
  Memory1 : Memory
  Memory2 : Memory
  TankModel : Subsystem
  LL1 : Outport
  wires:
  TankModel/1(LiquidLevel) -> Memory/1, LL1/1
  Control/1(LiquidIn) -> Logical Operator/1
  Control/2(LiquidOut) -> TankModel/2(LiquidOut)
  Memory/1 -> Control/5(LiquidLevel), MasterTankControl/1(LiquidTank1)
  MR1/1 -> Control/3(ManualReference)
  CT1/1 -> Control/2(StartMaintenance), Control/1(ControlType)
  LL3/1 -> Memory2/1
  Memory2/1 -> MasterTankControl/3(LiquidTank3)
  Memory1/1 -> MasterTankControl/2(LiquidTank2)
  EB1/1 -> Control/4(EmergencyButton)
  MasterTankControl/1(AllowTheTankFilling) -> Logical Operator/2
  Logical Operator/1 -> TankModel/1(LiquidIn)
  LL2/1 -> Memory1/1

== system c00011M_harness/M222/Tank2 ==
  CT2 : Inport
  MR2 : Inport  Port=2
  T2 : Inport  Port=3
  EB2 : Inport  Port=4
  LL1 : Inport  Port=5
  LL3 : Inport  Port=6
  Control : Subsystem
  Logical Operator : Logic  AllPortsSameDT=off  OutDataTypeStr=boolean
  MasterTankControl : Subsystem
  Memory : Memory
  Memory1 : Memory
  Memory2 : Memory
  TankModel : Subsystem
  LL2 : Outport
  wires:
  TankModel/1(LiquidLevel) -> Memory/1, LL2/1
  Control/1(LiquidIn) -> Logical Operator/1
  Control/2(LiquidOut) -> TankModel/2(LiquidOut)
  Memory/1 -> Control/5(LiquidLevel), MasterTankControl/2(LiquidTank2)
  MR2/1 -> Control/3(ManualReference)
  CT2/1 -> Control/2(StartMaintenance), Control/1(ControlType)
  LL3/1 -> Memory2/1
  Memory2/1 -> MasterTankControl/3(LiquidTank3)
  Memory1/1 -> MasterTankControl/1(LiquidTank1)
  EB2/1 -> Control/4(EmergencyButton)
  MasterTankControl/1(AllowTheTankFilling) -> Logical Operator/2
  Logical Operator/1 -> TankModel/1(LiquidIn)
  LL1/1 -> Memory1/1

== system c00011M_harness/M222/Tank3 ==
  CT3 : Inport
  F3 : Inport  Port=2
  E3 : Inport  Port=3
  T3 : Inport  Port=4
  EB3 : Inport  Port=5
  LL1 : Inport  Port=6
  LL2 : Inport  Port=7
  Control : Subsystem
  Logical Operator : Logic  AllPortsSameDT=off  OutDataTypeStr=boolean
  MasterTankControl : Subsystem
  Memory : Memory
  Memory1 : Memory
  Memory2 : Memory
  TankModel : Subsystem
  LL3 : Outport
  wires:
  TankModel/1(LiquidLevel) -> Memory/1, LL3/1
  Control/1(LiquidIn) -> Logical Operator/1
  Control/2(LiquidOut) -> TankModel/2(LiquidOut)
  Memory/1 -> MasterTankControl/3(LiquidTank3), Control/5(LiquidLevel)
  CT3/1 -> Control/1(ControlType)
  F3/1 -> Control/2(Fill)
  E3/1 -> Control/3(Empty)
  LL2/1 -> Memory2/1
  Memory2/1 -> MasterTankControl/2(LiquidTank2)
  Memory1/1 -> MasterTankControl/1(LiquidTank1)
  EB3/1 -> Control/4(EmergencyButton)
  MasterTankControl/1(AllowTheTankFilling) -> Logical Operator/2
  Logical Operator/1 -> TankModel/1(LiquidIn)
  LL1/1 -> Memory1/1

== system c00011M_harness/M223/Tank1 ==
  CT1 : Inport
  MR1 : Inport  Port=2
  T1 : Inport  Port=3
  EB1 : Inport  Port=4
  LL2 : Inport  Port=5
  LL3 : Inport  Port=6
  Control : Subsystem
  Logical Operator : Logic  AllPortsSameDT=off  OutDataTypeStr=boolean
  MasterTankControl : Subsystem
  Memory : Memory
  Memory1 : Memory
  Memory2 : Memory
  TankModel : Subsystem
  LL1 : Outport
  wires:
  TankModel/1(LiquidLevel) -> Memory/1, LL1/1
  Control/1(LiquidIn) -> Logical Operator/1
  Control/2(LiquidOut) -> TankModel/2(LiquidOut)
  Memory/1 -> Control/5(LiquidLevel), MasterTankControl/1(LiquidTank1)
  MR1/1 -> Control/3(ManualReference)
  CT1/1 -> Control/2(StartMaintenance), Control/1(ControlType)
  LL3/1 -> Memory2/1
  Memory2/1 -> MasterTankControl/3(LiquidTank3)
  Memory1/1 -> MasterTankControl/2(LiquidTank2)
  EB1/1 -> Control/4(EmergencyButton)
  MasterTankControl/1(AllowTheTankFilling) -> Logical Operator/2
  Logical Operator/1 -> TankModel/1(LiquidIn)
  LL2/1 -> Memory1/1

== system c00011M_harness/M223/Tank2 ==
  CT2 : Inport
  MR2 : Inport  Port=2
  T2 : Inport  Port=3
  EB2 : Inport  Port=4
  LL1 : Inport  Port=5
  LL3 : Inport  Port=6
  Control : Subsystem
  Logical Operator : Logic  AllPortsSameDT=off  OutDataTypeStr=boolean
  MasterTankControl : Subsystem
  Memory : Memory
  Memory1 : Memory
  Memory2 : Memory
  TankModel : Subsystem
  LL2 : Outport
  wires:
  TankModel/1(LiquidLevel) -> Memory/1, LL2/1
  Control/1(LiquidIn) -> Logical Operator/1
  Control/2(LiquidOut) -> TankModel/2(LiquidOut)
  Memory/1 -> Control/5(LiquidLevel), MasterTankControl/2(LiquidTank2)
  MR2/1 -> Control/3(ManualReference)
  CT2/1 -> Control/2(StartMaintenance), Control/1(ControlType)
  LL3/1 -> Memory2/1
  Memory2/1 -> MasterTankControl/3(LiquidTank3)
  Memory1/1 -> MasterTankControl/1(LiquidTank1)
  EB2/1 -> Control/4(EmergencyButton)
  MasterTankControl/1(AllowTheTankFilling) -> Logical Operator/2
  Logical Operator/1 -> TankModel/1(LiquidIn)
  LL1/1 -> Memory1/1

== system c00011M_harness/M223/Tank3 ==
  CT3 : Inport
  F3 : Inport  Port=2
  E3 : Inport  Port=3
  T3 : Inport  Port=4
  EB3 : Inport  Port=5
  LL1 : Inport  Port=6
  LL2 : Inport  Port=7
  Control : Subsystem
  Logical Operator : Logic  AllPortsSameDT=off  OutDataTypeStr=boolean
  MasterTankControl : Subsystem
  Memory : Memory
  Memory1 : Memory
  Memory2 : Memory
  TankModel : Subsystem
  LL3 : Outport
  wires:
  TankModel/1(LiquidLevel) -> Memory/1, LL3/1
  Control/1(LiquidIn) -> Logical Operator/1
  Control/2(LiquidOut) -> TankModel/2(LiquidOut)
  Memory/1 -> MasterTankControl/3(LiquidTank3), Control/5(LiquidLevel)
  CT3/1 -> Control/1(ControlType)
  F3/1 -> Control/2(Fill)
  E3/1 -> Control/3(Empty)
  LL2/1 -> Memory2/1
  Memory2/1 -> MasterTankControl/2(LiquidTank2)
  Memory1/1 -> MasterTankControl/1(LiquidTank1)
  EB3/1 -> Control/4(EmergencyButton)
  MasterTankControl/1(AllowTheTankFilling) -> Logical Operator/2
  Logical Operator/1 -> TankModel/1(LiquidIn)
  LL1/1 -> Memory1/1

== system c00011M_harness/M224/Tank1 ==
  CT1 : Inport
  MR1 : Inport  Port=2
  T1 : Inport  Port=3
  EB1 : Inport  Port=4
  LL2 : Inport  Port=5
  LL3 : Inport  Port=6
  Control : Subsystem
  Logical Operator : Logic  AllPortsSameDT=off  OutDataTypeStr=boolean
  MasterTankControl : Subsystem
  Memory : Memory
  Memory1 : Memory
  Memory2 : Memory
  TankModel : Subsystem
  LL1 : Outport
  wires:
  TankModel/1(LiquidLevel) -> Memory/1, LL1/1
  Control/1(LiquidIn) -> Logical Operator/1
  Control/2(LiquidOut) -> TankModel/2(LiquidOut)
  Memory/1 -> Control/5(LiquidLevel), MasterTankControl/1(LiquidTank1)
  MR1/1 -> Control/3(ManualReference)
  CT1/1 -> Control/2(StartMaintenance), Control/1(ControlType)
  LL3/1 -> Memory2/1
  Memory2/1 -> MasterTankControl/3(LiquidTank3)
  Memory1/1 -> MasterTankControl/2(LiquidTank2)
  EB1/1 -> Control/4(EmergencyButton)
  MasterTankControl/1(AllowTheTankFilling) -> Logical Operator/2
  Logical Operator/1 -> TankModel/1(LiquidIn)
  LL2/1 -> Memory1/1

== system c00011M_harness/M224/Tank2 ==
  CT2 : Inport
  MR2 : Inport  Port=2
  T2 : Inport  Port=3
  EB2 : Inport  Port=4
  LL1 : Inport  Port=5
  LL3 : Inport  Port=6
  Control : Subsystem
  Logical Operator : Logic  AllPortsSameDT=off  OutDataTypeStr=boolean
  MasterTankControl : Subsystem
  Memory : Memory
  Memory1 : Memory
  Memory2 : Memory
  TankModel : Subsystem
  LL2 : Outport
  wires:
  TankModel/1(LiquidLevel) -> Memory/1, LL2/1
  Control/1(LiquidIn) -> Logical Operator/1
  Control/2(LiquidOut) -> TankModel/2(LiquidOut)
  Memory/1 -> Control/5(LiquidLevel), MasterTankControl/2(LiquidTank2)
  MR2/1 -> Control/3(ManualReference)
  CT2/1 -> Control/2(StartMaintenance), Control/1(ControlType)
  LL3/1 -> Memory2/1
  Memory2/1 -> MasterTankControl/3(LiquidTank3)
  Memory1/1 -> MasterTankControl/1(LiquidTank1)
  EB2/1 -> Control/4(EmergencyButton)
  MasterTankControl/1(AllowTheTankFilling) -> Logical Operator/2
  Logical Operator/1 -> TankModel/1(LiquidIn)
  LL1/1 -> Memory1/1

== system c00011M_harness/M224/Tank3 ==
  CT3 : Inport
  F3 : Inport  Port=2
  E3 : Inport  Port=3
  T3 : Inport  Port=4
  EB3 : Inport  Port=5
  LL1 : Inport  Port=6
  LL2 : Inport  Port=7
  Control : Subsystem
  Logical Operator : Logic  AllPortsSameDT=off  OutDataTypeStr=boolean
  MasterTankControl : Subsystem
  Memory : Memory
  Memory1 : Memory
  Memory2 : Memory
  TankModel : Subsystem
  LL3 : Outport
  wires:
  TankModel/1(LiquidLevel) -> Memory/1, LL3/1
  Control/1(LiquidIn) -> Logical Operator/1
  Control/2(LiquidOut) -> TankModel/2(LiquidOut)
  Memory/1 -> MasterTankControl/3(LiquidTank3), Control/5(LiquidLevel)
  CT3/1 -> Control/1(ControlType)
  F3/1 -> Control/2(Fill)
  E3/1 -> Control/3(Empty)
  LL2/1 -> Memory2/1
  Memory2/1 -> MasterTankControl/2(LiquidTank2)
  Memory1/1 -> MasterTankControl/1(LiquidTank1)
  EB3/1 -> Control/4(EmergencyButton)
  MasterTankControl/1(AllowTheTankFilling) -> Logical Operator/2
  Logical Operator/1 -> TankModel/1(LiquidIn)
  LL1/1 -> Memory1/1

== system c00011M_harness/M225/Tank1 ==
  CT1 : Inport
  MR1 : Inport  Port=2
  T1 : Inport  Port=3
  EB1 : Inport  Port=4
  LL2 : Inport  Port=5
  LL3 : Inport  Port=6
  Control : Subsystem
  Logical Operator : Logic  AllPortsSameDT=off  OutDataTypeStr=boolean
  MasterTankControl : Subsystem
  Memory : Memory
  Memory1 : Memory
  Memory2 : Memory
  TankModel : Subsystem
  LL1 : Outport
  wires:
  TankModel/1(LiquidLevel) -> Memory/1, LL1/1
  Control/1(LiquidIn) -> Logical Operator/1
  Control/2(LiquidOut) -> TankModel/2(LiquidOut)
  Memory/1 -> Control/5(LiquidLevel), MasterTankControl/1(LiquidTank1)
  MR1/1 -> Control/3(ManualReference)
  CT1/1 -> Control/2(StartMaintenance), Control/1(ControlType)
  LL3/1 -> Memory2/1
  Memory2/1 -> MasterTankControl/3(LiquidTank3)
  Memory1/1 -> MasterTankControl/2(LiquidTank2)
  EB1/1 -> Control/4(EmergencyButton)
  MasterTankControl/1(AllowTheTankFilling) -> Logical Operator/2
  Logical Operator/1 -> TankModel/1(LiquidIn)
  LL2/1 -> Memory1/1

== system c00011M_harness/M225/Tank2 ==
  CT2 : Inport
  MR2 : Inport  Port=2
  T2 : Inport  Port=3
  EB2 : Inport  Port=4
  LL1 : Inport  Port=5
  LL3 : Inport  Port=6
  Control : Subsystem
  Logical Operator : Logic  AllPortsSameDT=off  OutDataTypeStr=boolean
  MasterTankControl : Subsystem
  Memory : Memory
  Memory1 : Memory
  Memory2 : Memory
  TankModel : Subsystem
  LL2 : Outport
  wires:
  TankModel/1(LiquidLevel) -> Memory/1, LL2/1
  Control/1(LiquidIn) -> Logical Operator/1
  Control/2(LiquidOut) -> TankModel/2(LiquidOut)
  Memory/1 -> Control/5(LiquidLevel), MasterTankControl/2(LiquidTank2)
  MR2/1 -> Control/3(ManualReference)
  CT2/1 -> Control/2(StartMaintenance), Control/1(ControlType)
  LL3/1 -> Memory2/1
  Memory2/1 -> MasterTankControl/3(LiquidTank3)
  Memory1/1 -> MasterTankControl/1(LiquidTank1)
  EB2/1 -> Control/4(EmergencyButton)
  MasterTankControl/1(AllowTheTankFilling) -> Logical Operator/2
  Logical Operator/1 -> TankModel/1(LiquidIn)
  LL1/1 -> Memory1/1

== system c00011M_harness/M225/Tank3 ==
  CT3 : Inport
  F3 : Inport  Port=2
  E3 : Inport  Port=3
  T3 : Inport  Port=4
  EB3 : Inport  Port=5
  LL1 : Inport  Port=6
  LL2 : Inport  Port=7
  Control : Subsystem
  Logical Operator : Logic  AllPortsSameDT=off  OutDataTypeStr=boolean
  MasterTankControl : Subsystem
  Memory : Memory
  Memory1 : Memory
  Memory2 : Memory
  TankModel : Subsystem
  LL3 : Outport
  wires:
  TankModel/1(LiquidLevel) -> Memory/1, LL3/1
  Control/1(LiquidIn) -> Logical Operator/1
  Control/2(LiquidOut) -> TankModel/2(LiquidOut)
  Memory/1 -> MasterTankControl/3(LiquidTank3), Control/5(LiquidLevel)
  CT3/1 -> Control/1(ControlType)
  F3/1 -> Control/2(Fill)
  E3/1 -> Control/3(Empty)
  LL2/1 -> Memory2/1
  Memory2/1 -> MasterTankControl/2(LiquidTank2)
  Memory1/1 -> MasterTankControl/1(LiquidTank1)
  EB3/1 -> Control/4(EmergencyButton)
  MasterTankControl/1(AllowTheTankFilling) -> Logical Operator/2
  Logical Operator/1 -> TankModel/1(LiquidIn)
  LL1/1 -> Memory1/1

== system c00011M_harness/M226/Tank1 ==
  CT1 : Inport
  MR1 : Inport  Port=2
  T1 : Inport  Port=3
  EB1 : Inport  Port=4
  LL2 : Inport  Port=5
  LL3 : Inport  Port=6
  Control : Subsystem
  Logical Operator : Logic  AllPortsSameDT=off  OutDataTypeStr=boolean
  MasterTankControl : Subsystem
  Memory : Memory
  Memory1 : Memory
  Memory2 : Memory
  TankModel : Subsystem
  LL1 : Outport
  wires:
  TankModel/1(LiquidLevel) -> Memory/1, LL1/1
  Control/1(LiquidIn) -> Logical Operator/1
  Control/2(LiquidOut) -> TankModel/2(LiquidOut)
  Memory/1 -> Control/5(LiquidLevel), MasterTankControl/1(LiquidTank1)
  MR1/1 -> Control/3(ManualReference)
  CT1/1 -> Control/2(StartMaintenance), Control/1(ControlType)
  LL3/1 -> Memory2/1
  Memory2/1 -> MasterTankControl/3(LiquidTank3)
  Memory1/1 -> MasterTankControl/2(LiquidTank2)
  EB1/1 -> Control/4(EmergencyButton)
  MasterTankControl/1(AllowTheTankFilling) -> Logical Operator/2
  Logical Operator/1 -> TankModel/1(LiquidIn)
  LL2/1 -> Memory1/1

== system c00011M_harness/M226/Tank2 ==
  CT2 : Inport
  MR2 : Inport  Port=2
  T2 : Inport  Port=3
  EB2 : Inport  Port=4
  LL1 : Inport  Port=5
  LL3 : Inport  Port=6
  Control : Subsystem
  Logical Operator : Logic  AllPortsSameDT=off  OutDataTypeStr=boolean
  MasterTankControl : Subsystem
  Memory : Memory
  Memory1 : Memory
  Memory2 : Memory
  TankModel : Subsystem
  LL2 : Outport
  wires:
  TankModel/1(LiquidLevel) -> Memory/1, LL2/1
  Control/1(LiquidIn) -> Logical Operator/1
  Control/2(LiquidOut) -> TankModel/2(LiquidOut)
  Memory/1 -> Control/5(LiquidLevel), MasterTankControl/2(LiquidTank2)
  MR2/1 -> Control/3(ManualReference)
  CT2/1 -> Control/2(StartMaintenance), Control/1(ControlType)
  LL3/1 -> Memory2/1
  Memory2/1 -> MasterTankControl/3(LiquidTank3)
  Memory1/1 -> MasterTankControl/1(LiquidTank1)
  EB2/1 -> Control/4(EmergencyButton)
  MasterTankControl/1(AllowTheTankFilling) -> Logical Operator/2
  Logical Operator/1 -> TankModel/1(LiquidIn)
  LL1/1 -> Memory1/1

== system c00011M_harness/M226/Tank3 ==
  CT3 : Inport
  F3 : Inport  Port=2
  E3 : Inport  Port=3
  T3 : Inport  Port=4
  EB3 : Inport  Port=5
  LL1 : Inport  Port=6
  LL2 : Inport  Port=7
  Control : Subsystem
  Logical Operator : Logic  Operator=OR  AllPortsSameDT=off  OutDataTypeStr=boolean
  MasterTankControl : Subsystem
  Memory : Memory
  Memory1 : Memory
  Memory2 : Memory
  TankModel : Subsystem
  LL3 : Outport
  wires:
  TankModel/1(LiquidLevel) -> Memory/1, LL3/1
  Control/1(LiquidIn) -> Logical Operator/1
  Control/2(LiquidOut) -> TankModel/2(LiquidOut)
  Memory/1 -> MasterTankControl/3(LiquidTank3), Control/5(LiquidLevel)
  CT3/1 -> Control/1(ControlType)
  F3/1 -> Control/2(Fill)
  E3/1 -> Control/3(Empty)
  LL2/1 -> Memory2/1
  Memory2/1 -> MasterTankControl/2(LiquidTank2)
  Memory1/1 -> MasterTankControl/1(LiquidTank1)
  EB3/1 -> Control/4(EmergencyButton)
  MasterTankControl/1(AllowTheTankFilling) -> Logical Operator/2
  Logical Operator/1 -> TankModel/1(LiquidIn)
  LL1/1 -> Memory1/1
